simulink model "TF_ex1"  (R2021b)
settings: Solver=VariableStepAuto  StartTime=0.0  StopTime=10.0  RelTol=1e-3
values from neighbouring files (symbols this model uses):
  den = [1 5]    [Transfer_Functions.m]
  num = [1 3]    [Transfer_Functions.m]
settings Model: Creator=Pedro Carrinho  LastModifiedBy=Leonardo
settings SolverCC: MaxConsecutiveMinStep=1000  AlgebraicLoopSolver=TrustRegion
settings DataIOCC: Refine=10000
settings DebuggingCC: SFMachineParentedDataDiag=warning

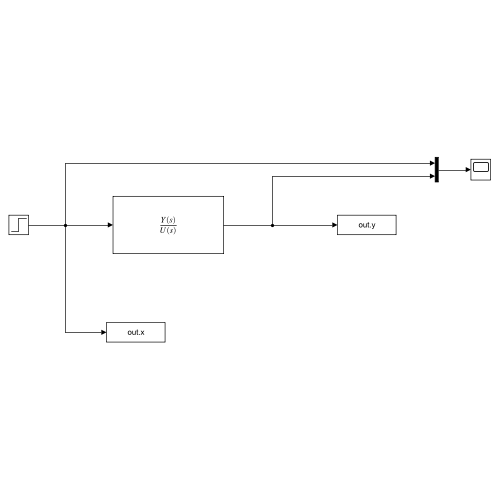
[thumbnail: Simulink's stored preview of the top-level diagram]
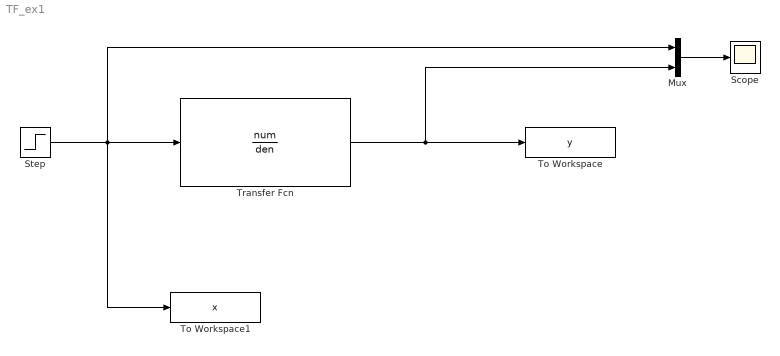
== system TF_ex1 ==
  Mux : Mux  Inputs=2
  Scope : Scope
  Step : Step  SampleTime=0
  To Workspace : ToWorkspace  VariableName=y  SaveFormat=Structure With Time  SampleTime=-1
  To Workspace1 : ToWorkspace  VariableName=x  SaveFormat=Structure With Time  SampleTime=-1
  Transfer Fcn : TransferFcn  Numerator=num  Denominator=den
  wires:
  Mux/1 -> Scope/1
  Transfer Fcn/1 -> To Workspace/1, Mux/2
  Step/1 -> To Workspace1/1, Mux/1, Transfer Fcn/1
